simulink model "merge_control_test"  (Simulink 8.2)
settings: Solver=ode1  StartTime=0.0  StopTime=Inf  FixedStep=0.001  RelTol=1e-3
PostLoadFcn:
  | , if any(exist('dsrtsu_mdlpostloadfcn', 'file') == [2, 3, 6]), try dsrtsu_mdlpostloadfcn('Execute', bdroot); catch fprintf('Error in PostLoadFcn (dsrtsu_mdlpostloadfcn) for model "%s":\n %s\n', bdroot, lasterr); end, end,
libraries: merge_control_lib x2
settings Model: DataTypeOverride=Double  MinMaxOverflowLogging=ForceOff  DSRTSU_INTERNAL_RTI_VER=450  DSRTSU_INTERNAL_RTI_TYPE=rti1401  DSRTSU_INTERNAL_RTIFPGA=40  Creator=rushk1  LastModifiedBy=rushk1  BufferReuse=off
settings DataIOCC: SignalLoggingSaveFormat=Dataset
settings OptimizationCC: BlockReduction=off  OptimizeBlockIOStorage=off  BufferReuse=off  ExpressionFolding=off  ExpressionDepthLimit=128  LocalBlockOutputs=off
settings DebuggingCC: FcnCallInpInsideContextMsg=EnableAllAsError  StateNameClashWarn=none
settings HardwareCC: TargetHWDeviceType=Generic->Custom
settings RTWCC: SystemTargetFile=rti1401.tlc  MakeCommand=make_rti  TemplateMakefile=rti1401.tmf  Description=dSPACE DS1401 Hardware Platform  ProcessScript=rti1401_make_rtw_hook
settings STFCustomTargetCC: CodeReplacementLibrary=ANSI_C  ParMdlRefBuildCompliant=on  GeneratePreprocessorConditionals=Disable all  MatFileLogging=on  SystemTargetFile=rti1401.tlc
settings GRTTargetCC: CompOptLevelCompliant=off  ConcurrentExecutionCompliant=off  ExtModeMexFile=noextcomm
settings CustomProperty: DataType=RTWOptions_EnumType_C__Program Files_dSPACE RCPHIL 2014-B_MATLAB_RTI_RTI1401_TLC_rti1401_1InitialSimState  Value=RUN
settings EnumStrPairs: String=RUN

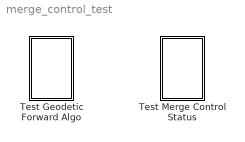
== system merge_control_test ==
  Test Geodetic Forward Algo : Subsystem
  Test Merge Control Status : Subsystem

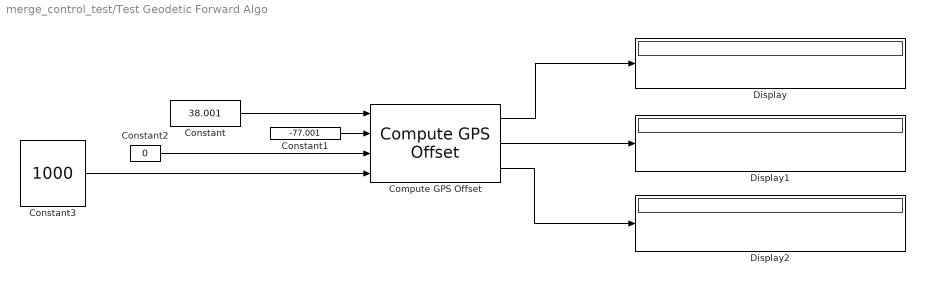
== system merge_control_test/Test Geodetic Forward Algo ==
  Compute GPS Offset : merge_control_lib/Compute GPS Offset
  Constant : Constant  Value=38.001
  Constant1 : Constant  Value=-77.001
  Constant2 : Constant  Value=0
  Constant3 : Constant  Value=1000
  Display : Display
      settings: Decimation=1000
  Display1 : Display
      settings: Decimation=1000
  Display2 : Display
  wires:
  Constant/1 -> Compute GPS Offset/1
  Constant1/1 -> Compute GPS Offset/2
  Constant2/1 -> Compute GPS Offset/3
  Constant3/1 -> Compute GPS Offset/4
  Compute GPS Offset/1 -> Display/1
  Compute GPS Offset/3 -> Display2/1
  Compute GPS Offset/2 -> Display1/1

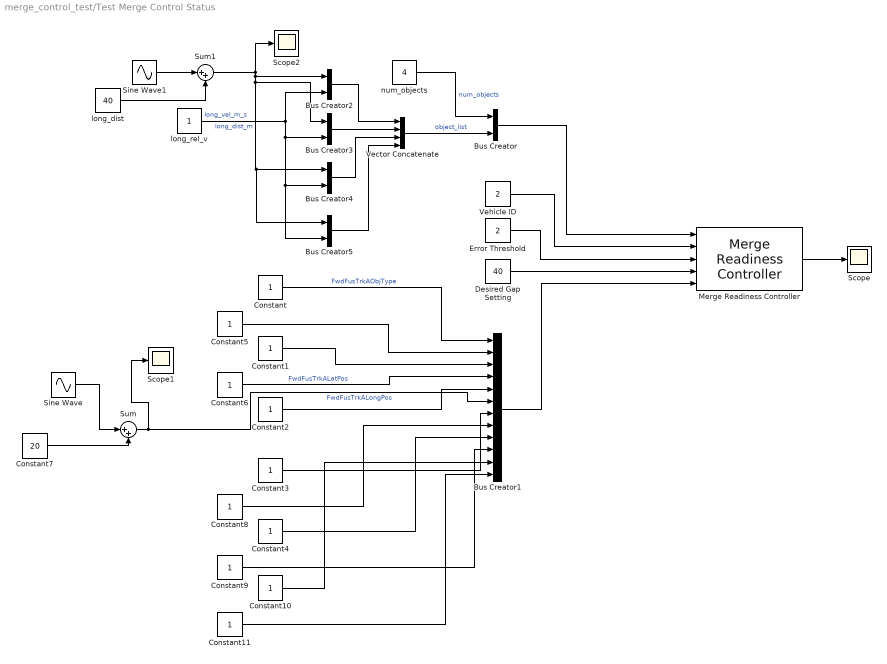
== system merge_control_test/Test Merge Control Status ==
  Bus Creator : BusCreator  Inputs=2  OutDataTypeStr=Bus: FusObjectList  NonVirtualBus=on
  Bus Creator1 : BusCreator  Inputs=12  OutDataTypeStr=Bus: FusObjectTrackA  NonVirtualBus=on
  Bus Creator{2..5} (4 alike) : BusCreator  Inputs=2  OutDataTypeStr=Bus: FusObjectData  NonVirtualBus=on
  Constant{,1..6,8..11} (11 alike) : Constant
  Constant7 : Constant  Value=20
  Desired Gap Setting : Constant  Value=40
  Error Threshold : Constant  Value=2
  Merge Readiness Controller : merge_control_lib/Merge Readiness Controller
  Scope : Scope
  Scope1 : Scope
      settings: YMin=15  YMax=25
  Scope2 : Scope
      settings: YMin=35  YMax=45  SaveName=ScopeData2
  Sine Wave : Sin  Amplitude=5  SampleTime=0
  Sine Wave1 : Sin  Amplitude=5  Frequency=.5  SampleTime=0
  Sum : Sum  Inputs=|++
  Sum1 : Sum  Inputs=|++
  Vector Concatenate : Concatenate  NumInputs=4
  Vehicle ID : Constant  Value=2
  long_dist : Constant  Value=40
  long_rel_v : Constant
  num_objects : Constant  Value=4  OutDataTypeStr=Inherit: Inherit via back propagation
  wires:
  Vehicle ID/1 -> Merge Readiness Controller/2
  Error Threshold/1 -> Merge Readiness Controller/3
  Bus Creator/1 -> Merge Readiness Controller/1
  Bus Creator1/1 -> Merge Readiness Controller/5
  Desired Gap Setting/1 -> Merge Readiness Controller/4
  Merge Readiness Controller/1 -> Scope/1
  Vector Concatenate/1 -> Bus Creator/2  "object_list"
  num_objects/1 -> Bus Creator/1  "num_objects"
  Bus Creator2/1 -> Vector Concatenate/1
  Bus Creator3/1 -> Vector Concatenate/2
  Bus Creator5/1 -> Vector Concatenate/4
  long_rel_v/1 -> Bus Creator2/2, Bus Creator5/2, Bus Creator4/2, Bus Creator3/2  "long_vel_m_s"
  Constant5/1 -> Bus Creator1/2
  Constant/1 -> Bus Creator1/1  "FwdFusTrkAObjType"
  Constant1/1 -> Bus Creator1/3
  Constant6/1 -> Bus Creator1/4  "FwdFusTrkALatPos"
  Constant2/1 -> Bus Creator1/5
  Constant3/1 -> Bus Creator1/7
  Constant8/1 -> Bus Creator1/8
  Constant4/1 -> Bus Creator1/9
  Constant9/1 -> Bus Creator1/10
  Constant10/1 -> Bus Creator1/11
  Constant11/1 -> Bus Creator1/12
  Bus Creator4/1 -> Vector Concatenate/3
  Sine Wave/1 -> Sum/1
  Constant7/1 -> Sum/2
  Sum/1 -> Scope1/1, Bus Creator1/6  "FwdFusTrkALongPos"
  long_dist/1 -> Sum1/2
  Sine Wave1/1 -> Sum1/1
  Sum1/1 -> Bus Creator5/1, Bus Creator4/1, Bus Creator3/1, Bus Creator2/1, Scope2/1  "long_dist_m"
